simulink model "Lab3"  (R2023a)
settings: Solver=VariableStepAuto  StartTime=0.0  StopTime=15  RelTol=1e-3
settings Model: Creator=Lenovo  LastModifiedBy=Lenovo

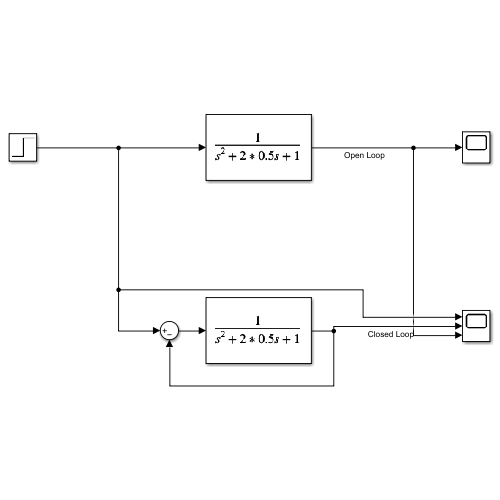
[thumbnail: Simulink's stored preview of the top-level diagram]
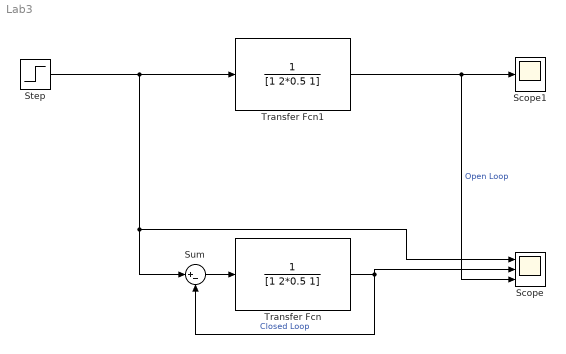
== system Lab3 ==
  Scope : Scope  NumInputPorts=3
  Scope1 : Scope
  Step : Step  SampleTime=0
  Sum : Sum  Inputs=|+-
  Transfer Fcn : TransferFcn  Denominator=[1 2*0.5 1]
  Transfer Fcn1 : TransferFcn  Denominator=[1 2*0.5 1]
  wires:
  Transfer Fcn/1 -> Scope/2, Sum/2  "Closed Loop"
  Step/1 -> Scope/1, Sum/1, Transfer Fcn1/1
  Sum/1 -> Transfer Fcn/1
  Transfer Fcn1/1 -> Scope/3, Scope1/1  "Open Loop"
